simulink library "VsrLibHilUtils"  (R2019b)
settings: Solver=VariableStepAuto  StartTime=0.0  StopTime=10.0  RelTol=1e-3
libraries: simulink x2
settings Model: Creator=9bt  LastModifiedBy=admin

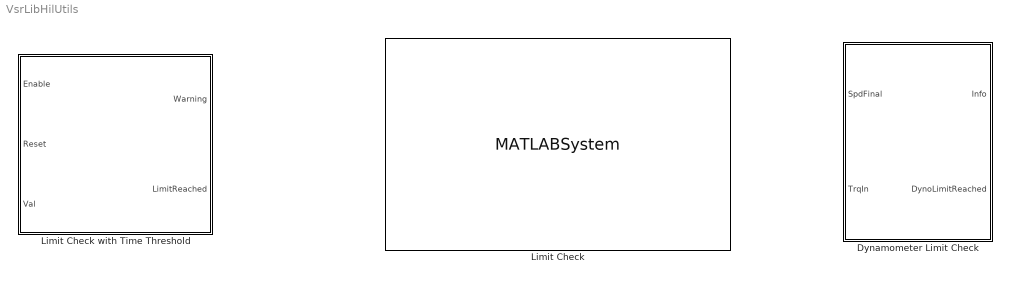
== system VsrLibHilUtils ==
  Dynamometer Limit Check : Subsystem  mask{NumDynos=1, DynoSpdMax=5000*pi/30, DynoGearRatio=2.611, DynoTrqMaxSpdBpts=linspace(0,550, 25), DynoTrqMaxTbl=min(3750, 500e3./linspace(0,550, 25))}
      mask prompts: NumDynos "Number of dynamometers connected in parallel:"; DynoSpdMax "Maximum dynamometer speed, DynoSpdMax [rad/s]:"; DynoGearRatio "Dynamometer gear ratio, DynoGearRatio []:"; DynoTrqMaxSpdBpts "Dynamometer max torque table speed breakpoints, DynoTrqMaxSpdBpts [rad/s]:"; DynoTrqMaxTbl "Dynamometer max torque table, DynoTrqMaxTbl [rad/s]:"
      mask help: Block determines if dynamometer reaches torque or speed limits based on simulated test scenario.
      mask TypeOptions NumDynos: 1 | 2
  Limit Check : MATLABSystem  System=vsr.hil.HilLimitSystemBlock  OutputTbls=true  ValueNames=[123,39,120,32,49,39,44,39,121,39,44,39,122,39,44,39,120,50,39,44,39,120,51,39,125]  LowerLimit=[1;nan;nan;nan;nan]  LowerWarning=[3;nan;nan;nan;nan]  UpperWarning=[nan;nan;nan;nan;nan]  UpperLimit=[nan;nan;nan;nan;nan]  SimulateUsing=Code generation
      settings: OpenFcn=|
      | app = VsrLimitBlockUI;
      | app.updateBlockDialog(gcb);
      mask Type: vsr.hil.HilLimitSystemBlock
      mask Display:
      | disp('vsr.hil.HilLimitSystemBlock');
      | port_label('input',1,'Enable');
      | port_label('input',2,'Reset');
      | port_label('input',3,'Port1');
      | port_label('input',4,'Port2');
      | port_label('input',5,'Port3');
      | port_label('input',6,'Port4');
      | port_label('input',7,'Port5');
      | port_label('output',1,'Warning');
      | port_label('output',2,'LimitReached');
      | port_label('output',3,'WarningTbl');
      | port_label('output',4,'LimitReachedTbl');
      | port_label('output',5,'ValTbl');
      | port_label('output',6,'ValMinTbl');
      | port_label('output',7,'ValMaxTbl');
  Limit Check with Time Threshold : Subsystem  mask{CheckLowerLimit=on, CheckUpperLimit=on, Unit=inherit, LowerWarning=0, LowerWarningTime=0, LowerLimit=0, LowerLimitTime=0, UpperWarning=0, UpperWarningTime=0, UpperLimit=0, UpperLimitTime=0}
      mask prompts: CheckLowerLimit "Check lower limit"; CheckUpperLimit "Check upper limit"; Unit "Simulink:blkprm_prompts:OutputUnit_EditField"; LowerWarning "Lower warning:"; LowerWarningTime "Lower warning time:"; LowerLimit "Lower limit:"; LowerLimitTime "Lower limit time:"; UpperWarning "Upper warning:"; UpperWarningTime "Upper warning time:"; UpperLimit "Upper limit:"; UpperLimitTime "Upper limit time"
      mask TypeOptions Unit: Signal Specification/Unit
      mask DialogControl Unit Prompt: Unit (e.g., m, m/s^2, N*m):
      mask DialogControl Container3 Prompt: Lower Limit
      mask DialogControl Container4 Prompt: Upper Limit

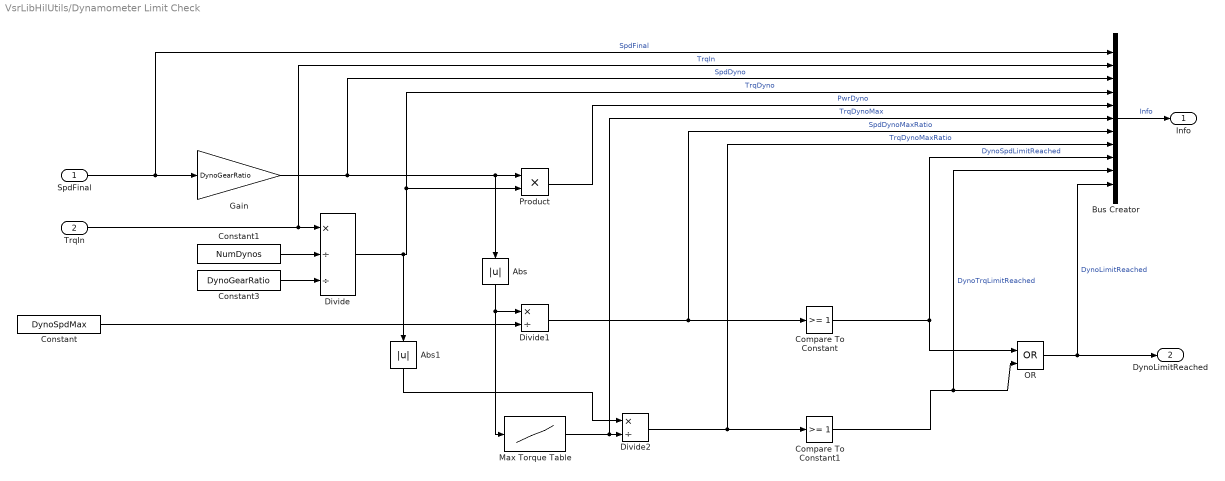
== system VsrLibHilUtils/Dynamometer Limit Check ==
  SpdFinal : Inport  Unit=rad/s
  TrqIn : Inport  Port=2  Unit=N*m
  Abs : Abs  ZeroCross=off
  Abs1 : Abs  ZeroCross=off
  Bus Creator : BusCreator  Inputs=11
  Compare To Constant : simulink/Logic and Bit Operations/Compare To Constant  relop=>=  const=1  OutDataTypeStr=boolean  ZeroCross=off
  Compare To Constant1 : simulink/Logic and Bit Operations/Compare To Constant  relop=>=  const=1  OutDataTypeStr=boolean  ZeroCross=off
  Constant : Constant  Value=DynoSpdMax
  Constant1 : Constant  Value=NumDynos
  Constant3 : Constant  Value=DynoGearRatio
  Divide : Product  Inputs=*//
  Divide1 : Product  Inputs=*/
  Divide2 : Product  Inputs=*/
  Gain : Gain  Gain=DynoGearRatio
  Max Torque Table : Lookup_n-D  NumberOfTableDimensions=1  BreakpointsForDimension1=DynoTrqMaxSpdBpts  Table=DynoTrqMaxTbl  ExtrapMethod=Clip  InternalRulePriority=Speed  RndMeth=Simplest  InputSameDT=on
  OR : Logic  Operator=OR  IconShape=distinctive  AllPortsSameDT=off  OutDataTypeStr=boolean
  Product : Product
  Info : Outport
  DynoLimitReached : Outport  Port=2
  wires:
  SpdFinal/1 -> Bus Creator/1, Gain/1  "SpdFinal"
  Gain/1 -> Abs/1, Product/1, Bus Creator/3  "SpdDyno"
  TrqIn/1 -> Bus Creator/2, Divide/1  "TrqIn"
  Constant1/1 -> Divide/2
  Constant3/1 -> Divide/3
  Divide/1 -> Bus Creator/4, Product/2, Abs1/1  "TrqDyno"
  Product/1 -> Bus Creator/5  "PwrDyno"
  Abs1/1 -> Divide2/1
  Max Torque Table/1 -> Bus Creator/6, Divide2/2  "TrqDynoMax"
  Divide1/1 -> Compare To Constant/1, Bus Creator/7  "SpdDynoMaxRatio"
  Divide2/1 -> Compare To Constant1/1, Bus Creator/8  "TrqDynoMaxRatio"
  Bus Creator/1 -> Info/1  "Info"
  Compare To Constant/1 -> OR/1, Bus Creator/9  "DynoSpdLimitReached"
  Compare To Constant1/1 -> OR/2, Bus Creator/10  "DynoTrqLimitReached"
  OR/1 -> Bus Creator/11, DynoLimitReached/1  "DynoLimitReached"
  Constant/1 -> Divide1/2
  Abs/1 -> Max Torque Table/1, Divide1/1

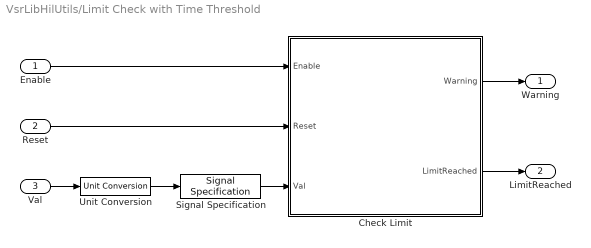
== system VsrLibHilUtils/Limit Check with Time Threshold ==
  Enable : Inport
  Reset : Inport  Port=2
  Val : Inport  Port=3
  Check Limit : Stateflow chart  BlockKeywords=__PRM__SERIALIZED__DATA__:Stateflow Chart,Stateflow Diagram  TreatAsAtomicUnit=on
  Signal Specification : SignalSpecification
  Unit Conversion : UnitConversion
  Warning : Outport
  LimitReached : Outport  Port=2
  wires:
  Enable/1 -> Check Limit/1(Enable)
  Reset/1 -> Check Limit/2(Reset)
  Val/1 -> Unit Conversion/1
  Check Limit/2(LimitReached) -> LimitReached/1
  Check Limit/1(Warning) -> Warning/1
  Signal Specification/1 -> Check Limit/3(Val)
  Unit Conversion/1 -> Signal Specification/1

== stateflow chart VsrLibHilUtils/Limit Check with Time Threshold/Check Limit ==
  state LimitCheckEnabled
    state LowerWarningCheck [parallel]
      settings: executionOrder=1
      state WarningValReached
      state LowerWarningActive
      state WarningNotReached
      (default) -> LimitCheckEnabled.LowerWarningCheck.WarningNotReached
      LimitCheckEnabled.LowerWarningCheck.WarningNotReached -> LimitCheckEnabled.LowerWarningCheck.WarningValReached : [CheckLowerLimit && ...
          | Val <= LowerWarning]
      LimitCheckEnabled.LowerWarningCheck.WarningValReached -> LowerWarningActive [order 2] : after(LowerWarningTime, sec)
      LimitCheckEnabled.LowerWarningCheck.WarningValReached -> LimitCheckEnabled.LowerWarningCheck.WarningNotReached [order 1] : [Val > LowerWarning]
      LowerWarningActive -> LimitCheckEnabled.LowerWarningCheck.WarningValReached : [Val > LowerWarning]
    state LowerLimitCheck [parallel]
      settings: executionOrder=2
      state LimitValReached
      state LowerLimitActive
      state LimitNotReached
      (default) -> LimitCheckEnabled.LowerLimitCheck.LimitNotReached
      LimitCheckEnabled.LowerLimitCheck.LimitNotReached -> LimitCheckEnabled.LowerLimitCheck.LimitValReached : [CheckLowerLimit && ...
          | Val <= LowerLimit]
      LimitCheckEnabled.LowerLimitCheck.LimitValReached -> LowerLimitActive [order 2] : after(LowerLimitTime, sec)
      LimitCheckEnabled.LowerLimitCheck.LimitValReached -> LimitCheckEnabled.LowerLimitCheck.LimitNotReached [order 1] : [Val > LowerLimit]
      LowerLimitActive -> LimitCheckEnabled.LowerLimitCheck.LimitValReached : [Reset]
    state UpperWarningCheck [parallel]
      settings: executionOrder=3
      state WarningValReached
      state UpperWarningActive
      state WarningNotReached
      (default) -> LimitCheckEnabled.UpperWarningCheck.WarningNotReached
      LimitCheckEnabled.UpperWarningCheck.WarningNotReached -> LimitCheckEnabled.UpperWarningCheck.WarningValReached : [CheckUpperLimit && ...
          | Val >= UpperWarning]
      LimitCheckEnabled.UpperWarningCheck.WarningValReached -> UpperWarningActive [order 2] : after(UpperWarningTime, sec)
      LimitCheckEnabled.UpperWarningCheck.WarningValReached -> LimitCheckEnabled.UpperWarningCheck.WarningNotReached [order 1] : [Val < UpperWarning]
      UpperWarningActive -> LimitCheckEnabled.UpperWarningCheck.WarningValReached : [Val < UpperWarning]
    state UpperLimitCheck [parallel]
      settings: executionOrder=4
      state LimitValReached
      state UpperLimitActive
      state LimitNotReached
      (default) -> LimitCheckEnabled.UpperLimitCheck.LimitNotReached
      LimitCheckEnabled.UpperLimitCheck.LimitNotReached -> LimitCheckEnabled.UpperLimitCheck.LimitValReached : [CheckUpperLimit && ...
          | Val >= UpperLimit]
      LimitCheckEnabled.UpperLimitCheck.LimitValReached -> UpperLimitActive [order 2] : after(UpperLimitTime, sec)
      LimitCheckEnabled.UpperLimitCheck.LimitValReached -> LimitCheckEnabled.UpperLimitCheck.LimitNotReached [order 1] : [Val < UpperLimit]
      UpperLimitActive -> LimitCheckEnabled.UpperLimitCheck.LimitValReached : [Reset]
    state LimitUpdate [parallel]
      du: Warning = in(LowerWarningCheck.LowerWarningActive) || in(UpperWarningCheck.UpperWarningActive);
      LimitReached = in(LowerLimitCheck.LowerLimitActive) || in(UpperLimitCheck.UpperLimitActive);
      settings: executionOrder=5
  state LimitCheckDisable
    en:
    Warning = false;
    LimitReached = false;
  (default) -> LimitCheckDisable : {Warning = false;
      | LimitReached = false;}
  LimitCheckDisable -> LimitCheckEnabled : [Enable]
  LimitCheckEnabled -> LimitCheckDisable : [~Enable]
  data: Enable input boolean; Reset input boolean; Warning output; LimitReached output; Val input; LowerWarning parameter; LowerLimitTime parameter; LowerLimit parameter; LowerWarningTime parameter; CheckLowerLimit parameter; CheckUpperLimit parameter; UpperLimitTime parameter; UpperLimit parameter; UpperWarningTime parameter; UpperWarning parameter
